simulink model "LiPo_Plant"  (R2022b)
settings: Solver=ode15s  StartTime=0.0  StopTime=5  FixedStep=1e-5  MaxStep=1e-3  RelTol=1e-3
undefined symbols (not defined in the file or in its folder): Bat, ESC, fan, LookUp, motor
libraries: slpidlib x1
settings Model: Creator=User  LastModifiedBy=User

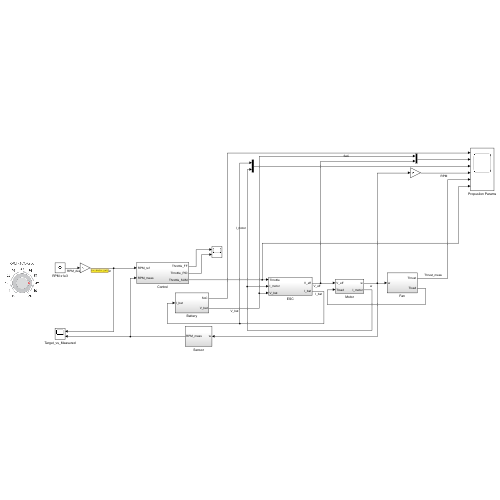
[thumbnail: Simulink's stored preview of the top-level diagram]
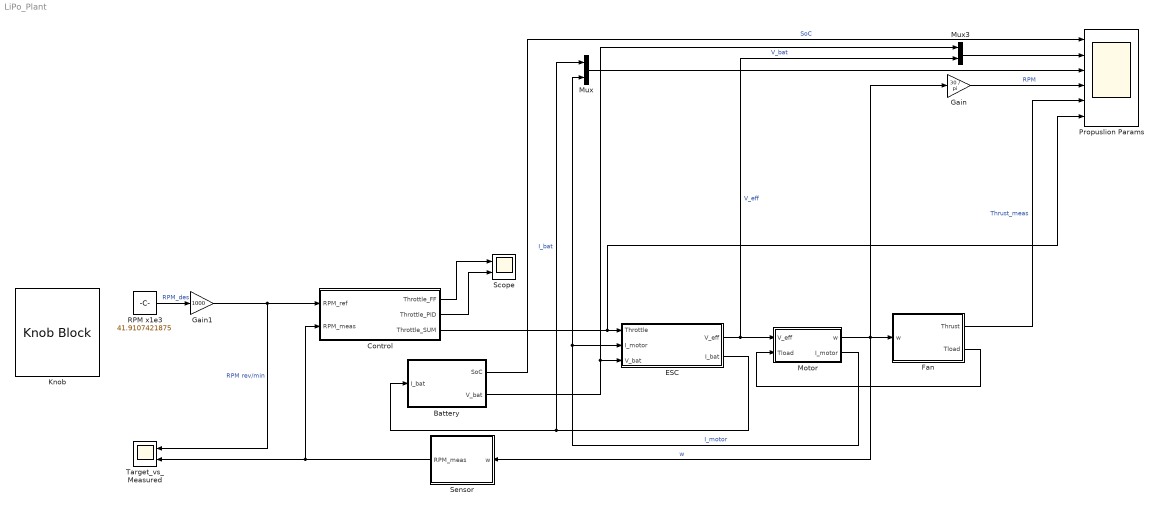
== system LiPo_Plant ==
  Battery : Subsystem
  Control : Subsystem
  ESC : Subsystem
  Fan : Subsystem
  Gain : Gain  Gain=30 / pi
  Gain1 : Gain  Gain=1000
  Knob : KnobBlock  ScaleMin=10  ScaleMax=50
  Motor : Subsystem
  Mux : Mux  Inputs=2
  Mux3 : Mux  Inputs=2
  Propuslion Params : Scope  NumInputPorts=6
  RPM x1e3 : Constant  Value=41.9107421875
  Scope : Scope  NumInputPorts=2
  Sensor : Subsystem
  Target_vs_Measured : Scope  NumInputPorts=2
  wires:
  Battery/2(V_bat) -> Mux3/1, ESC/3(V_bat)  "V_bat"
  ESC/2(I_bat) -> Battery/1(I_bat), Mux/1  "I_bat"
  Motor/1(w) -> Sensor/1(w), Gain/1, Fan/1(w)  "w"
  Motor/2(I_motor) -> Mux/2, ESC/2(I_motor)  "I_motor"
  ESC/1(V_eff) -> Mux3/2, Motor/1(V_eff)  "V_eff"
  Fan/1(Thrust) -> Propuslion Params/5  "Thrust_meas"
  Battery/1(SoC) -> Propuslion Params/1  "SoC"
  Mux/1 -> Propuslion Params/3
  Gain/1 -> Propuslion Params/4  "RPM"
  Fan/2(Tload) -> Motor/2(Tload)
  Gain1/1 -> Target_vs_Measured/1, Control/1(RPM_ref)  "RPM rev/min"
  Sensor/1(RPM_meas) -> Control/2(RPM_meas), Target_vs_Measured/2
  RPM x1e3/1 -> Gain1/1  "RPM_des"
  Mux3/1 -> Propuslion Params/2
  Control/3(Throttle_SUM) -> Propuslion Params/6, ESC/1(Throttle)
  Control/1(Throttle_FF) -> Scope/1
  Control/2(Throttle_PID) -> Scope/2

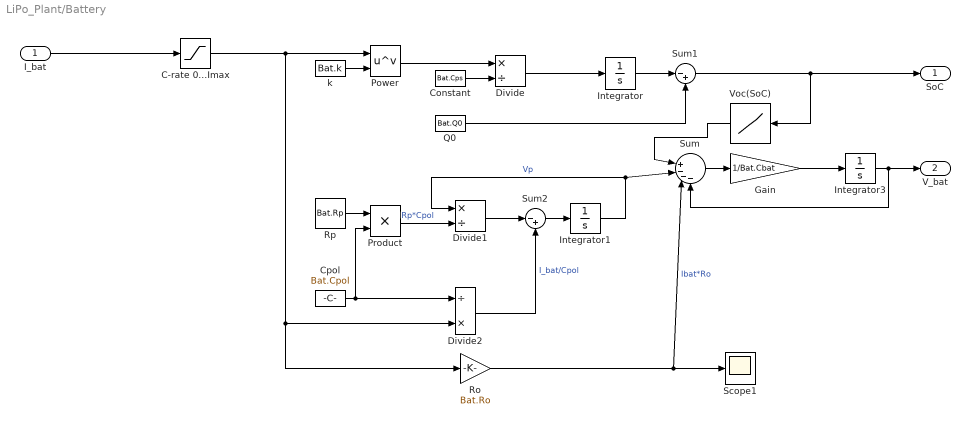
== system LiPo_Plant/Battery ==
  I_bat : Inport
  C-rate 0...Imax : Saturate  UpperLimit=Bat.Imax  LowerLimit=0
  Constant : Constant  Value=Bat.Cps
  Cpol : Constant  Value=Bat.Cpol
  Divide : Product  Inputs=*/
  Divide1 : Product  Inputs=*/
  Divide2 : Product  Inputs=/*
  Gain : Gain  Gain=1/Bat.Cbat
  Integrator : Integrator
  Integrator1 : Integrator
  Integrator3 : Integrator  InitialCondition=Bat.Vcell*Bat.ncell
  Power : Math  Operator=pow
  Product : Product
  Q0 : Constant  Value=Bat.Q0
  Ro : Gain  Gain=Bat.Ro
  Rp : Constant  Value=Bat.Rp
  Scope1 : Scope
  Sum : Sum  Inputs=||+---
  Sum1 : Sum  Inputs=|-+
  Sum2 : Sum  Inputs=|-+
  Voc(SoC) : Lookup_n-D  NumberOfTableDimensions=1  BreakpointsForDimension1=LookUp.SoC  Table=LookUp.Volts  InternalRulePriority=Speed  RndMeth=Simplest
  k : Constant  Value=Bat.k
  SoC : Outport
  V_bat : Outport  Port=2
  wires:
  Integrator1/1 -> Divide1/1, Sum/2  "Vp"
  Sum2/1 -> Integrator1/1
  Product/1 -> Divide1/2  "Rp*Cpol"
  Q0/1 -> Sum1/2
  Cpol/1 -> Divide2/1, Product/2
  Voc(SoC)/1 -> Sum/1
  Rp/1 -> Product/1
  Power/1 -> Divide/1
  Constant/1 -> Divide/2
  k/1 -> Power/2
  Sum/1 -> Gain/1
  I_bat/1 -> C-rate 0...Imax/1
  Integrator/1 -> Sum1/1
  Sum1/1 -> Voc(SoC)/1, SoC/1
  Divide1/1 -> Sum2/1
  Divide2/1 -> Sum2/2  "I_bat/Cpol"
  Ro/1 -> Sum/3, Scope1/1  "Ibat*Ro"
  Divide/1 -> Integrator/1
  C-rate 0...Imax/1 -> Ro/1, Divide2/2, Power/1
  Integrator3/1 -> Sum/4, V_bat/1
  Gain/1 -> Integrator3/1

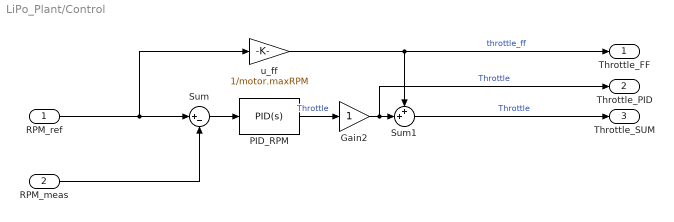
== system LiPo_Plant/Control ==
  RPM_ref : Inport
  RPM_meas : Inport  Port=2
  Gain2 : Gain
  PID_RPM : slpidlib/PID Controller  Controller=PID  Form=Parallel  TimeDomain=Continuous-time  UseExternalTs=off  SampleTime=-1  IntegratorMethod=Forward Euler  FilterMethod=Forward Euler  ControllerParametersSource=internal  P=1e-4  I=0  UseKiTs=off  D=0  N=100  UseFilter=on  TunerSelectOption=Transfer Function Based (PID Tuner App)  InitialConditionSource=internal  InitialConditionForIntegrator=0  InitialConditionForFilter=0  DifferentiatorICPrevScaledInput=0  ExternalReset=none  TrackingMode=off  Kt=1  LimitOutput=on  SatLimitsSource=internal  UpperSaturationLimit=1  LowerSaturationLimit=0  LinearizeAsGain=on  AntiWindupMode=none  Kb=1  LimitIntegrator=off  UpperIntegratorSaturationLimit=inf  LowerIntegratorSaturationLimit=-inf  POutMin=[]  POutMax=[]  IOutMin=[]  IOutMax=[]  DOutMin=[]  DOutMax=[]  NOutMin=[]  NOutMax=[]  SumOutMin=[]  SumOutMax=[]  SaturationOutMin=[]  SaturationOutMax=[]  PParamMin=[]  PParamMax=[]  IParamMin=[]  IParamMax=[]  DParamMin=[]  DParamMax=[]  NParamMin=[]  NParamMax=[]  KbParamMin=[]  KbParamMax=[]  KtParamMin=[]  KtParamMax=[]  KbOutMin=[]  KbOutMax=[]  KtOutMin=[]  KtOutMax=[]  IntegratorOutMin=[]  IntegratorOutMax=[]  FilterOutMin=[]  FilterOutMax=[]  SumI1OutMin=[]  SumI1OutMax=[]  SumI2OutMin=[]  SumI2OutMax=[]  SumI3OutMin=[]  SumI3OutMax=[]  SumI4OutMin=[]  SumI4OutMax=[]  SumDOutMin=[]  SumDOutMax=[]  DifferentiatorOutMin=[]  DifferentiatorOutMax=[]  FilterDiffOutCoefMin=[]  FilterDiffOutCoefMax=[]  ReciprocalOutMin=[]  ReciprocalOutMax=[]  SumDenOutMin=[]  SumDenOutMax=[]  SumNumOutMin=[]  SumNumOutMax=[]  DivideOutMin=[]  DivideOutMax=[]  UdiffTsProdOutMin=[]  UdiffTsProdOutMax=[]  NTsProdOutMin=[]  NTsProdOutMax=[]  UintegralTsProdOutMin=[]  UintegralTsProdOutMax=[]  UngainTsProdOutMin=[]  UngainTsProdOutMax=[]  ClampingZeroOutDataTypeStr=Inherit: Inherit via back propagation  ClampingZeroOutMin=[]  ClampingZeroOutMax=[]  FilterDenConstantOutDataTypeStr=Inherit: Inherit via back propagation  FilterDenConstantOutMin=[]  FilterDenConstantOutMax=[]  PCopyOutDataTypeStr=Inherit: Inherit via back propagation  PCopyOutMin=[]  PCopyOutMax=[]  NCopyOutDataTypeStr=Inherit: Inherit via back propagation  NCopyOutMin=[]  NCopyOutMax=[]  IntegratorContinuousStateAttributes=''  IntegratorStateMustResolveToSignalObject=off  IntegratorRTWStateStorageClass=Auto  FilterContinuousStateAttributes=''  FilterStateMustResolveToSignalObject=off  FilterRTWStateStorageClass=Auto  ParallelPVariant=InternalParameters  IdealPVariant=Disabled  IVariant=InternalParameters  DVariant=InternalParameters  IntegratorVariant=Continuous  SatVariant=Enabled  AWVariant=Passthrough  PCopyVariant=Disabled  TRVariant=Disabled  FdbkBlocksVariant=Forward  IdealPFdbkVariant=Disabled  SatFdbkVariant=Disabled  DerivativeFilterVariant=ContFilter  NVariant=InternalParameters  NCopyVariant=Disabled  FilterICVariant=InternalICsFilter  IntegratorICVariant=InternalICs  ExternalResetVariant=Disabled  TRSumVariant=Passthrough  SumFdbkVariant=Disabled  SumVariant=Sum_PID  TsampFilterVariant=InternalTs  TsampNgainVariant=Passthrough  TsampIntegralVariant=Passthrough  ExternalSaturationOutDataTypeStr=Inherit: Same as second input
  Sum : Sum  Inputs=|+-
  Sum1 : Sum  Inputs=++|
  u_ff : Gain  Gain=1/motor.maxRPM
  Throttle_FF : Outport
  Throttle_PID : Outport  Port=2
  Throttle_SUM : Outport  Port=3
  wires:
  Sum1/1 -> Throttle_SUM/1  "Throttle"
  Gain2/1 -> Throttle_PID/1, Sum1/2  "Throttle"
  RPM_meas/1 -> Sum/2
  Sum/1 -> PID_RPM/1
  RPM_ref/1 -> Sum/1, u_ff/1
  u_ff/1 -> Sum1/1, Throttle_FF/1  "throttle_ff"
  PID_RPM/1 -> Gain2/1  "Throttle"

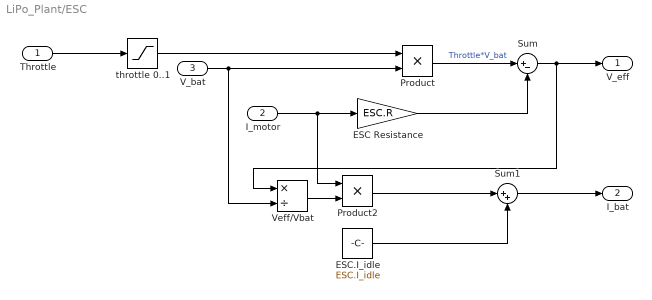
== system LiPo_Plant/ESC ==
  Throttle : Inport
  I_motor : Inport  Port=2
  V_bat : Inport  Port=3
  ESC Resistance : Gain  Gain=ESC.R
  ESC.I_idle : Constant  Value=ESC.I_idle
  Product : Product
  Product2 : Product
  Sum : Sum  Inputs=|+-
  Sum1 : Sum  Inputs=|++
  Veff/Vbat : Product  Inputs=*/
  throttle 0..1 : Saturate  UpperLimit=1  LowerLimit=0
  V_eff : Outport
  I_bat : Outport  Port=2
  wires:
  Throttle/1 -> throttle 0..1/1
  V_bat/1 -> Product/2, Veff/Vbat/2
  Product/1 -> Sum/1  "Throttle*V_bat"
  Sum1/1 -> I_bat/1
  ESC Resistance/1 -> Sum/2
  Sum/1 -> V_eff/1, Veff/Vbat/1
  I_motor/1 -> ESC Resistance/1, Product2/1
  Veff/Vbat/1 -> Product2/2
  Product2/1 -> Sum1/1
  ESC.I_idle/1 -> Sum1/2
  throttle 0..1/1 -> Product/1

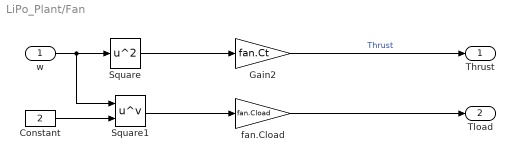
== system LiPo_Plant/Fan ==
  w : Inport
  Constant : Constant  Value=2
  Gain2 : Gain  Gain=fan.Ct
  Square : Math  Operator=square
  Square1 : Math  Operator=pow
  fan.Cload : Gain  Gain=fan.Cload
  Thrust : Outport
  Tload : Outport  Port=2
  wires:
  Square/1 -> Gain2/1
  Gain2/1 -> Thrust/1  "Thrust"
  w/1 -> Square1/1, Square/1
  Constant/1 -> Square1/2
  Square1/1 -> fan.Cload/1
  fan.Cload/1 -> Tload/1

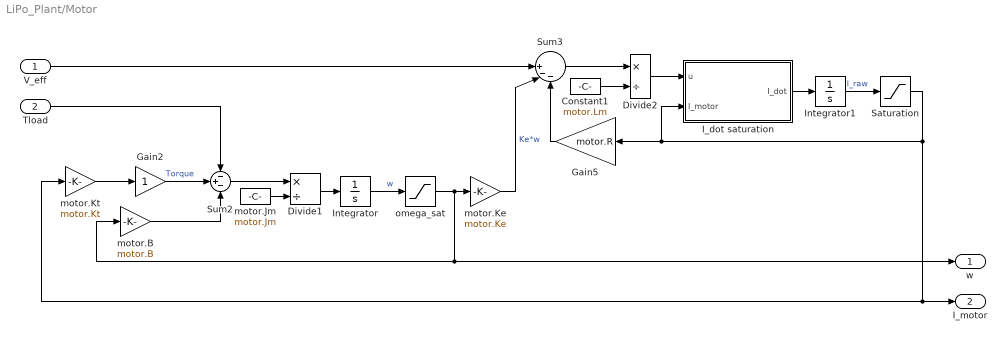
== system LiPo_Plant/Motor ==
  V_eff : Inport
  Tload : Inport  Port=2
  Constant1 : Constant  Value=motor.Lm
  Divide1 : Product  Inputs=*/
  Divide2 : Product  Inputs=*/
  Gain2 : Gain
  Gain5 : Gain  Gain=motor.R
  I_dot saturation : MATLAB Function  TreatAsAtomicUnit=on
  Integrator : Integrator
  Integrator1 : Integrator
  Saturation : Saturate  UpperLimit=motor.Imax  LowerLimit=-motor.Imax
  Sum2 : Sum  Inputs=-+-
  Sum3 : Sum  Inputs=||+--
  motor.B : Gain  Gain=motor.B
  motor.Jm : Constant  Value=motor.Jm
  motor.Ke : Gain  Gain=motor.Ke
  motor.Kt : Gain  Gain=motor.Kt
  omega_sat : Saturate  UpperLimit=motor.maxFreq  LowerLimit=0
  w : Outport
  I_motor : Outport  Port=2
  wires:
  motor.Jm/1 -> Divide1/2
  Divide1/1 -> Integrator/1
  motor.Kt/1 -> Gain2/1
  Integrator/1 -> omega_sat/1  "w"
  Constant1/1 -> Divide2/2
  motor.Ke/1 -> Sum3/2  "Ke*w"
  Integrator1/1 -> Saturation/1  "I_raw"
  V_eff/1 -> Sum3/1
  Gain2/1 -> Sum2/2  "Torque"
  Sum2/1 -> Divide1/1
  Tload/1 -> Sum2/1
  motor.B/1 -> Sum2/3
  Sum3/1 -> Divide2/1
  Gain5/1 -> Sum3/3
  Saturation/1 -> I_dot saturation/2(I_motor), Gain5/1, motor.Kt/1, I_motor/1
  Divide2/1 -> I_dot saturation/1(u)
  I_dot saturation/1(I_dot) -> Integrator1/1
  omega_sat/1 -> motor.B/1, w/1, motor.Ke/1

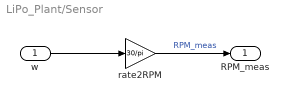
== system LiPo_Plant/Sensor ==
  w : Inport
  rate2RPM : Gain  Gain=30/pi
  RPM_meas : Outport
  wires:
  rate2RPM/1 -> RPM_meas/1  "RPM_meas"
  w/1 -> rate2RPM/1

== matlab function LiPo_Plant/Motor/I_dot saturation ==
  data: u input; I_dot output; I_motor input
function I_dot = Idot(u, I_motor)

% parameters (define as mask parameters or globals)
I_max = 120;     % example
u_max = 1e6;     % A/s, numerical safety limit

% guard against NaN / Inf
if ~isfinite(u)
    I_dot = 0;
    return;
end

% limit derivative (ESC bandwidth / numerical safety)
u = max(min(u, u_max), -u_max);

% saturation detection (NOT at zero!)
sat = abs(I_motor) >= I_max;

% pushing further only if current is nonzero
push = (I_motor ~= 0) && (sign(u) == sign(I_motor));

if sat && push
    I_dot = 0;
else
    I_dot = u;
end
